simulink model "Model"  (R2021b)
settings: Solver=ode4  StartTime=0.0  StopTime=10  FixedStep=.005  RelTol=1e-3
values from neighbouring files (symbols this model uses):
  h = 0.25    [HW9.m]
settings Model: Creator=17165  LastModifiedBy=17165

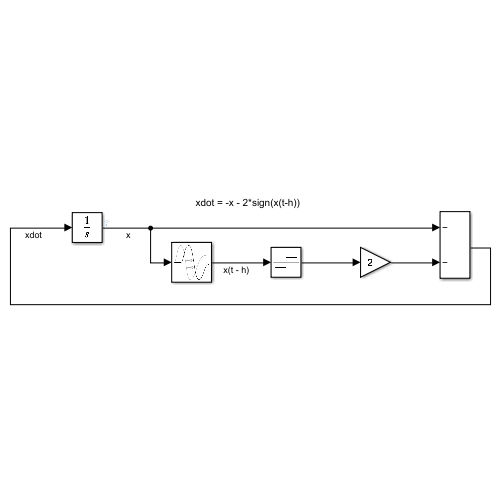
[thumbnail: Simulink's stored preview of the top-level diagram]
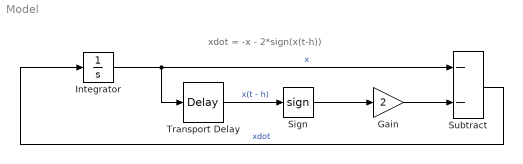
== system Model ==
  note: xdot = -x - 2*sign(x(t-h))
  Gain : Gain  Gain=2
  Integrator : Integrator  InitialCondition=2
  Sign : Signum
  Subtract : Sum  Inputs=--
  Transport Delay : TransportDelay  DelayTime=h
  wires:
  Sign/1 -> Gain/1
  Transport Delay/1 -> Sign/1  "x(t - h)"
  Integrator/1 -> Subtract/1, Transport Delay/1  "x"
  Gain/1 -> Subtract/2
  Subtract/1 -> Integrator/1  "xdot"
